simulink model "RL_Runcontrol_ruler"  (R2024b)
settings: Solver=VariableStepAuto  StartTime=0.0  StopTime=60  RelTol=1e-3
libraries: Solver_SF x1
settings Model: Creator=Administrator  LastModifiedBy=Administrator

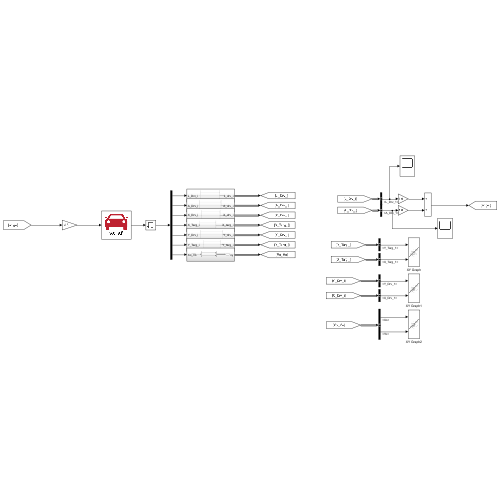
[thumbnail: Simulink's stored preview of the top-level diagram]
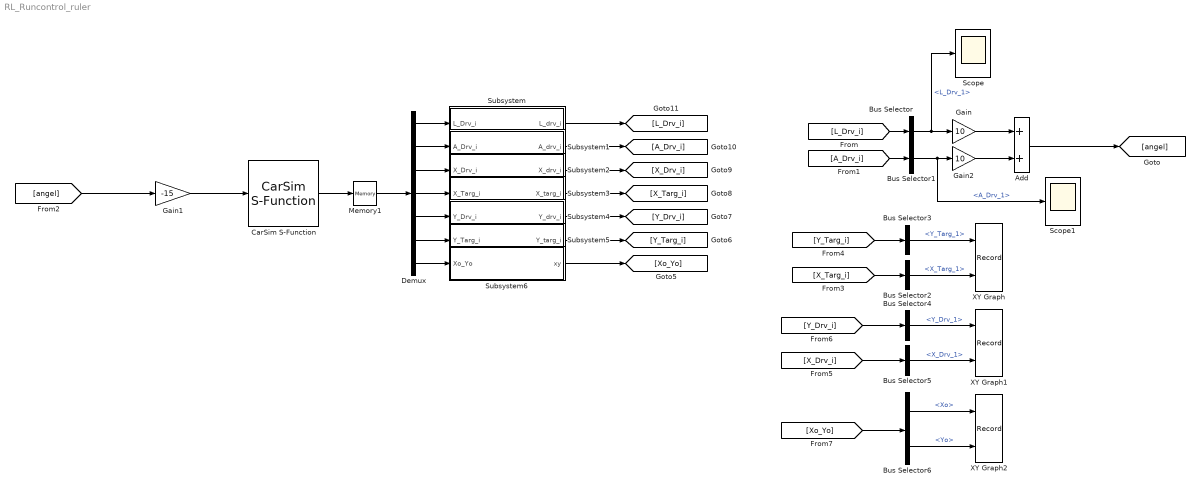
== system RL_Runcontrol_ruler ==
  Add : Sum
  Bus Selector : BusSelector  OutputSignals=L_Drv_1
  Bus Selector1 : BusSelector  OutputSignals=A_Drv_1
  Bus Selector2 : BusSelector  OutputSignals=X_Targ_1
  Bus Selector3 : BusSelector  OutputSignals=Y_Targ_1
  Bus Selector4 : BusSelector  OutputSignals=Y_Drv_1
  Bus Selector5 : BusSelector  OutputSignals=X_Drv_1
  Bus Selector6 : BusSelector  OutputSignals=Xo,Yo
  CarSim S-Function : Solver_SF/CarSim S-Function  Priority=1  SIMFILE=simfile.sim  Run_RTs=off  vs_state_ind=Run  StopMode_ind=Vehicle Model
  Demux : Demux  Outputs=[3 3 3 3 3 3 2]
  Gain : Gain  Gain=10
  Gain1 : Gain  Gain=-15
  Gain2 : Gain  Gain=10
  Memory1 : Memory
  Scope : Scope
  Scope1 : Scope
  Subsystem : Subsystem
  Subsystem1 : Subsystem
  Subsystem2 : Subsystem
  Subsystem3 : Subsystem
  Subsystem4 : Subsystem
  Subsystem5 : Subsystem
  Subsystem6 : Subsystem
  XY Graph : Record  FileSettingsInternal="{\"entries\":[{\"content\":{\"excelSettings\":{\"content\":{},\"type\":\"Streamout.ExcelSettings\"}},\"type\":\"Streamout.FileSettingStorage\",\"uuid\":\"\"}],\"packageUris\":[\"http:\\/\\/schema.mathworks.com\\/mf0\\/streamout_blocks\\/R2020a\"],\"version\":\"1.0\"}"  Layout=[1 1]  SignalsInternal="{\"entries\":[{\"content\":{},\"type\":\"RecordBlkView.InputSignals\",\"uuid\":\"\"}],\"packageUris\":[\"http:\\/\\/schema.mathworks.com\\/mf0\\/streamout_blocks\\/R2020a\"],\"version\":\"1.0\"}"  VisualizationBindings="{\"xyplotplugin\":{\"info\":[{\"series\":[{\"bindingParametersList\":[{\"parameter\":\"X-Axis\",\"signalID\":2585,\"signalName\":\"<Y_Targ_1>\"},{\"parameter\":\"Y-Axis\",\"signalID\":2589,\"signalName\":\"<X_Targ_1>\"}],\"seriesID\":0}],\"subplotID\":1}]}}"  CompatibilityTag=XY
  XY Graph1 : Record  FileSettingsInternal="{\"entries\":[{\"content\":{\"excelSettings\":{\"content\":{},\"type\":\"Streamout.ExcelSettings\"}},\"type\":\"Streamout.FileSettingStorage\",\"uuid\":\"\"}],\"packageUris\":[\"http:\\/\\/schema.mathworks.com\\/mf0\\/streamout_blocks\\/R2020a\"],\"version\":\"1.0\"}"  Layout=[1 1]  SignalsInternal="{\"entries\":[{\"content\":{},\"type\":\"RecordBlkView.InputSignals\",\"uuid\":\"\"}],\"packageUris\":[\"http:\\/\\/schema.mathworks.com\\/mf0\\/streamout_blocks\\/R2020a\"],\"version\":\"1.0\"}"  VisualizationBindings="{\"xyplotplugin\":{\"info\":[{\"series\":[{\"bindingParametersList\":[{\"parameter\":\"X-Axis\",\"signalID\":2593,\"signalName\":\"<Y_Drv_1>\"},{\"parameter\":\"Y-Axis\",\"signalID\":2597,\"signalName\":\"<X_Drv_1>\"}],\"seriesID\":0}],\"subplotID\":1}]}}"  CompatibilityTag=XY
  XY Graph2 : Record  FileSettingsInternal="{\"entries\":[{\"content\":{\"excelSettings\":{\"content\":{},\"type\":\"Streamout.ExcelSettings\"}},\"type\":\"Streamout.FileSettingStorage\",\"uuid\":\"\"}],\"packageUris\":[\"http:\\/\\/schema.mathworks.com\\/mf0\\/streamout_blocks\\/R2020a\"],\"version\":\"1.0\"}"  Layout=[1 1]  SignalsInternal="{\"entries\":[{\"content\":{\"signals\":[{\"content\":{\"blockPath\":[],\"dimensions\":[1],\"domain\":\"\",\"lineColor\":\"#a2142f\",\"port\":1,\"sid\":[\"\"],\"signalID\":1,\"signalName\":\"<Y_Targ_1>\"},\"type\":\"RecordBlkView.Signal\",\"uuid\":\"\"},{\"content\":{\"blockPath\":[],\"dimensions\":[1],\"domain\":\"\",\"lineColor\":\"#139fff\",\"port\":2,\"sid\":[\"\"],\"signalID\":2,\"signalName\":\"<X_Targ_1>\"},\"type\":\"RecordBlkView.Signal\",\"uuid\":\"\"},{\"content\":{\"blockPath\":[],\"dimensions\":[1],\"domain\":\"\",\"lineColor\":\"#a2142f\",\"port\":1,\"sid\":[\"\"],\"signalID\":3,\"signalName\":\"<Y_Drv_1>\"},\"type\":\"RecordBlkView.Signal\",\"uuid\":\"\"},{\"content\":{\"blockPath\":[],\"dimensions\":[1],\"domain\":\"\",\"lineColor\":\"#139fff\",\"port\":2,\"sid\":[\"\"],\"signalID\":4,\"signalName\":\"<X_Drv_1>\"},\"type\":\"RecordBlkView.Signal\",\"uuid\":\"\"},{\"content\":{\"blockPath\":[],\"dimensions\":[1],\"domain\":\"\",\"lineColor\":\"#a2142f\",\"plots\":[ 1 ],\"port\":1,\"sid\":[\"\"],\"signalID\":5,\"signalName\":\"<Xo>\"},\"type\":\"RecordBlkView.Signal\",\"uuid\":\"\"},{\"content\":{\"blockPath\":[],\"dimensions\":[1],\"domain\":\"\",\"lineColor\":\"#139fff\",\"plots\":[ 1 ],\"port\":2,\"sid\":[\"\"],\"signalID\":6,\"signalName\":\"<Yo>\"},\"type\":\"RecordBlkView.Signal\",\"uuid\":\"\"}]},\"type\":\"RecordBlkView.InputSignals\",\"uuid\":\"\"}],\"packageUris\":[\"http:\\/\\/schema.mathworks.com\\/mf0\\/streamout_blocks\\/R2020a\"],\"version\":\"1.0\"}"  VisualizationBindings="{\"xyplotplugin\":{\"info\":[{\"series\":[{\"bindingParametersList\":[{\"parameter\":\"X-Axis\",\"signalID\":5,\"signalName\":\"<Xo>\"},{\"parameter\":\"Y-Axis\",\"signalID\":6,\"signalName\":\"<Yo>\"}],\"seriesID\":0}],\"subplotID\":1}]}}"  CompatibilityTag=XY
  wires:
  CarSim S-Function/1 -> Memory1/1
  Memory1/1 -> Demux/1
  Demux/1 -> Subsystem/1(L_Drv_i)
  Demux/2 -> Subsystem1/1(A_Drv_i)
  Demux/3 -> Subsystem2/1(X_Drv_i)
  Demux/4 -> Subsystem3/1(X_Targ_i)
  Demux/5 -> Subsystem4/1(Y_Drv_i)
  Demux/6 -> Subsystem5/1(Y_Targ_i)
  Demux/7 -> Subsystem6/1(Xo_Yo)
  Subsystem/1(L_drv_i) -> [L_Drv_i]
  Subsystem1/1(A_drv_i) -> [A_Drv_i]
  Subsystem2/1(X_drv_i) -> [X_Drv_i]
  Subsystem3/1(X_targ_i) -> [X_Targ_i]
  Subsystem4/1(Y_drv_i) -> [Y_Drv_i]
  Subsystem5/1(Y_targ_i) -> [Y_Targ_i]
  Subsystem6/1(xy) -> [Xo_Yo]
  [L_Drv_i] -> Bus Selector/1
  [A_Drv_i] -> Bus Selector1/1
  Bus Selector/1 -> Scope/1, Gain/1  "<L_Drv_1>"
  Bus Selector1/1 -> Scope1/1, Gain2/1  "<A_Drv_1>"
  Gain/1 -> Add/1
  Add/1 -> [angel]
  [angel] -> Gain1/1
  [X_Targ_i] -> Bus Selector2/1
  [Y_Targ_i] -> Bus Selector3/1
  Bus Selector3/1 -> XY Graph/1  "<Y_Targ_1>"
  Bus Selector2/1 -> XY Graph/2  "<X_Targ_1>"
  [Y_Drv_i] -> Bus Selector4/1
  [X_Drv_i] -> Bus Selector5/1
  Bus Selector4/1 -> XY Graph1/1  "<Y_Drv_1>"
  Bus Selector5/1 -> XY Graph1/2  "<X_Drv_1>"
  Gain1/1 -> CarSim S-Function/1
  Gain2/1 -> Add/2
  [Xo_Yo] -> Bus Selector6/1
  Bus Selector6/1 -> XY Graph2/1  "<Xo>"
  Bus Selector6/2 -> XY Graph2/2  "<Yo>"

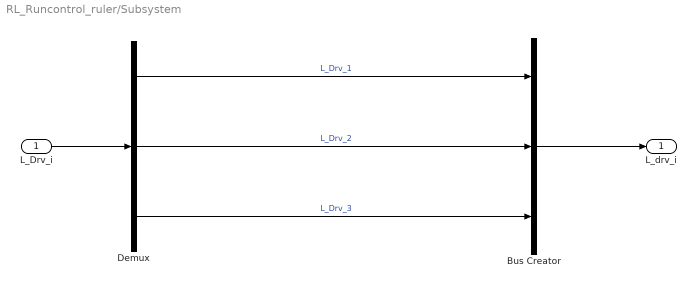
== system RL_Runcontrol_ruler/Subsystem ==
  L_Drv_i : Inport
  Bus Creator : BusCreator  Inputs=3
  Demux : Demux  Outputs=3
  L_drv_i : Outport
  wires:
  L_Drv_i/1 -> Demux/1
  Demux/1 -> Bus Creator/1  "L_Drv_1"
  Demux/2 -> Bus Creator/2  "L_Drv_2"
  Demux/3 -> Bus Creator/3  "L_Drv_3"
  Bus Creator/1 -> L_drv_i/1

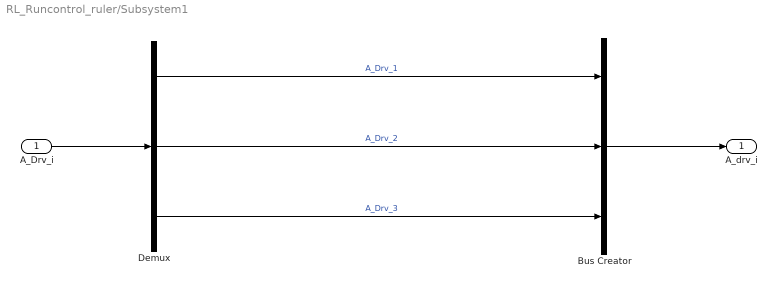
== system RL_Runcontrol_ruler/Subsystem1 ==
  A_Drv_i : Inport
  Bus Creator : BusCreator  Inputs=3
  Demux : Demux  Outputs=3
  A_drv_i : Outport
  wires:
  A_Drv_i/1 -> Demux/1
  Demux/3 -> Bus Creator/3  "A_Drv_3"
  Demux/1 -> Bus Creator/1  "A_Drv_1"
  Demux/2 -> Bus Creator/2  "A_Drv_2"
  Bus Creator/1 -> A_drv_i/1

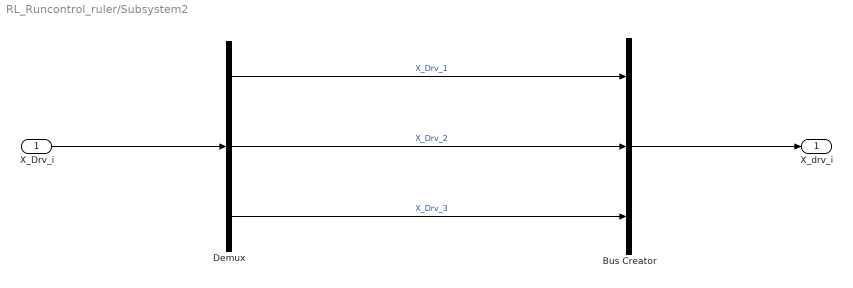
== system RL_Runcontrol_ruler/Subsystem2 ==
  X_Drv_i : Inport
  Bus Creator : BusCreator  Inputs=3
  Demux : Demux  Outputs=3
  X_drv_i : Outport
  wires:
  X_Drv_i/1 -> Demux/1
  Demux/3 -> Bus Creator/3  "X_Drv_3"
  Demux/1 -> Bus Creator/1  "X_Drv_1"
  Demux/2 -> Bus Creator/2  "X_Drv_2"
  Bus Creator/1 -> X_drv_i/1

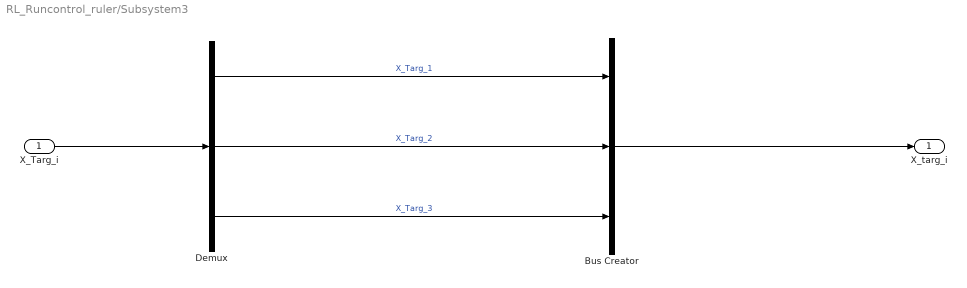
== system RL_Runcontrol_ruler/Subsystem3 ==
  X_Targ_i : Inport
  Bus Creator : BusCreator  Inputs=3
  Demux : Demux  Outputs=3
  X_targ_i : Outport
  wires:
  X_Targ_i/1 -> Demux/1
  Demux/3 -> Bus Creator/3  "X_Targ_3"
  Demux/1 -> Bus Creator/1  "X_Targ_1"
  Demux/2 -> Bus Creator/2  "X_Targ_2"
  Bus Creator/1 -> X_targ_i/1

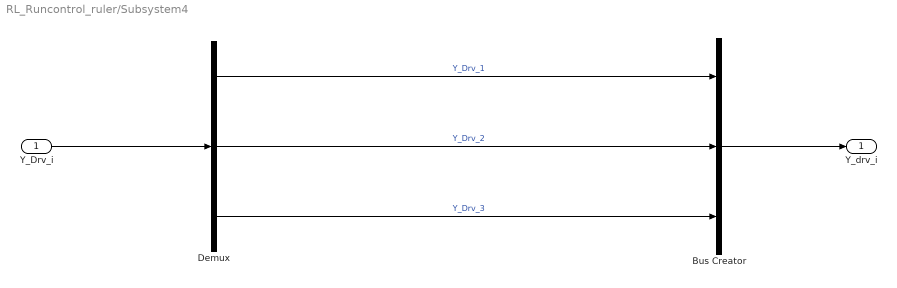
== system RL_Runcontrol_ruler/Subsystem4 ==
  Y_Drv_i : Inport
  Bus Creator : BusCreator  Inputs=3
  Demux : Demux  Outputs=3
  Y_drv_i : Outport
  wires:
  Y_Drv_i/1 -> Demux/1
  Demux/3 -> Bus Creator/3  "Y_Drv_3"
  Demux/1 -> Bus Creator/1  "Y_Drv_1"
  Demux/2 -> Bus Creator/2  "Y_Drv_2"
  Bus Creator/1 -> Y_drv_i/1

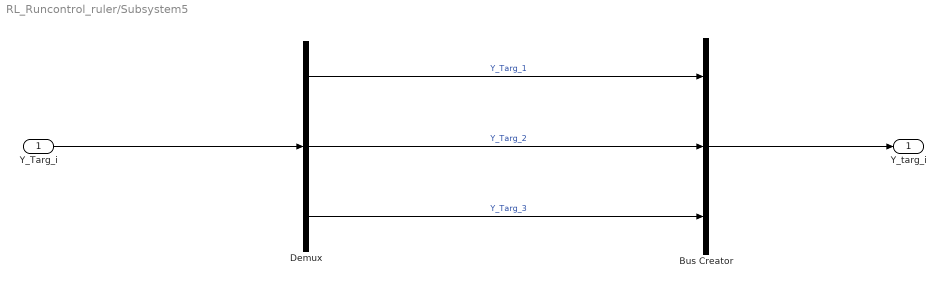
== system RL_Runcontrol_ruler/Subsystem5 ==
  Y_Targ_i : Inport
  Bus Creator : BusCreator  Inputs=3
  Demux : Demux  Outputs=3
  Y_targ_i : Outport
  wires:
  Y_Targ_i/1 -> Demux/1
  Demux/3 -> Bus Creator/3  "Y_Targ_3"
  Demux/1 -> Bus Creator/1  "Y_Targ_1"
  Demux/2 -> Bus Creator/2  "Y_Targ_2"
  Bus Creator/1 -> Y_targ_i/1

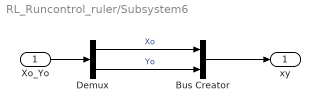
== system RL_Runcontrol_ruler/Subsystem6 ==
  Xo_Yo : Inport
  Bus Creator : BusCreator  Inputs=2
  Demux : Demux  Outputs=2
  xy : Outport
  wires:
  Xo_Yo/1 -> Demux/1
  Demux/1 -> Bus Creator/1  "Xo"
  Demux/2 -> Bus Creator/2  "Yo"
  Bus Creator/1 -> xy/1
